simulink model "altitude_from_pitch_loop"  (Simulink 9.0)
settings: Solver=VariableStepAuto  StartTime=0.0  StopTime=100  RelTol=1e-3
InitFcn:
  | param_chap6
values from neighbouring files (symbols this model uses):
  G = getGains(P,G)    [param_chap6.m]
libraries: cstblocks x2
settings Model: SuppressorTable=22 serialization::archive 11 0 6 0 0 0 0 0  Creator=leonardopedroso  LastModifiedBy=leonardopedroso
settings DataIOCC: SaveFormat=Dataset
settings OptimizationCC: LifeSpan=auto
settings DebuggingCC: UnderspecifiedInitializationDetection=Simplified  MergeDetectMultiDrivingBlocksExec=error  SFUnexpectedBacktrackingDiag=error  SFNoUnconditionalDefaultTransitionDiag=error  SFExecutionAtInitializationDiag=warning
settings HardwareCC: ProdBitPerPointer=64  ProdBitPerSizeT=64  ProdBitPerPtrDiffT=64  ProdLargestAtomicFloat=Float  ProdIntDivRoundTo=Zero  ProdEndianess=LittleEndian  ProdWordSize=64  ProdHWDeviceType=Intel->x86-64 (Windows64)
settings ModelReferenceCC: PropagateSignalLabelsOutOfModel=on
settings CodeAppCC: StateflowObjectComments=off
settings GRTTargetCC: TargetLangStandard=C99 (ISO)
settings ConfigComp: CovMetricSettings=dwe  CovHtmlReporting=off  CovSaveCumulativeToWorkspaceVar=off  CovSaveSingleToWorkspaceVar=off  CovExternalEMLEnable=on

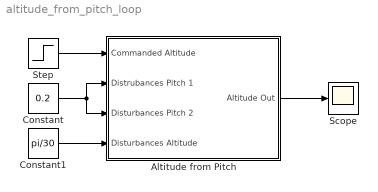
== system altitude_from_pitch_loop ==
  Altitude from Pitch : Subsystem
  Constant : Constant  Value=0.2
  Constant1 : Constant  Value=pi/30
  Scope : Scope
  Step : Step  Time=50  After=2  SampleTime=0
  wires:
  Altitude from Pitch/1(Altitude Out) -> Scope/1
  Constant/1 -> Altitude from Pitch/3(Disturbances Pitch 2), Altitude from Pitch/2(Distrubances Pitch 1)
  Constant1/1 -> Altitude from Pitch/4(Disturbances Altitude)
  Step/1 -> Altitude from Pitch/1(Commanded Altitude)

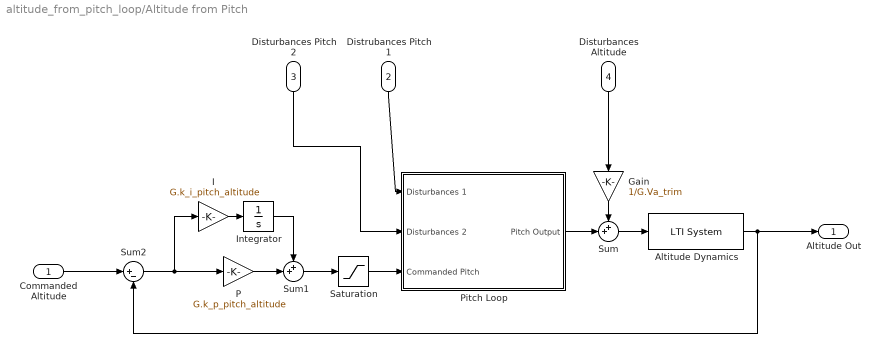
== system altitude_from_pitch_loop/Altitude from Pitch ==
  Commanded Altitude : Inport
  Distrubances Pitch 1 : Inport  Port=2
  Disturbances Pitch 2 : Inport  Port=3
  Disturbances Altitude : Inport  Port=4
  Altitude Dynamics : cstblocks/LTI System  sys=T_h_theta  IC=[]
  Gain : Gain  Gain=1/G.Va_trim
  I : Gain  Gain=G.k_i_pitch_altitude
  Integrator : Integrator
  P : Gain  Gain=G.k_p_pitch_altitude
  "Pitch Loop " : Subsystem
  Saturation : Saturate  UpperLimit=pi/4  LowerLimit=-pi/4
  Sum : Sum  Inputs=++|
  Sum1 : Sum  Inputs=++|
  Sum2 : Sum  Inputs=|+-
  Altitude Out : Outport
  wires:
  I/1 -> Integrator/1
  Sum/1 -> Altitude Dynamics/1
  Altitude Dynamics/1 -> Altitude Out/1, Sum2/2
  Integrator/1 -> Sum1/1
  P/1 -> Sum1/2
  "Pitch Loop "/1(Pitch Output) -> Sum/2
  Distrubances Pitch 1/1 -> "Pitch Loop "/1(Disturbances 1)
  Gain/1 -> Sum/1
  Sum2/1 -> P/1, I/1
  Commanded Altitude/1 -> Sum2/1
  Disturbances Pitch 2/1 -> "Pitch Loop "/2("Disturbances 2 ")
  Disturbances Altitude/1 -> Gain/1
  Sum1/1 -> Saturation/1
  Saturation/1 -> "Pitch Loop "/3(Commanded Pitch)

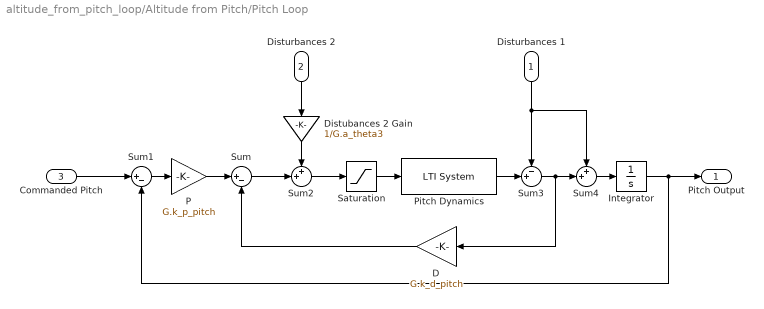
== system altitude_from_pitch_loop/Altitude from Pitch/Pitch Loop  ==
  Disturbances 1 : Inport
  "Disturbances 2 " : Inport  Port=2
  Commanded Pitch : Inport  Port=3
  D : Gain  Gain=G.k_d_pitch
  Distubances 2 Gain : Gain  Gain=1/G.a_theta3
  Integrator : Integrator
  "P " : Gain  Gain=G.k_p_pitch
  Pitch Dynamics : cstblocks/LTI System  sys=T_theta_dot_delta_e  IC=[]
  Saturation : Saturate  UpperLimit=G.delta_e_max  LowerLimit=-G.delta_a_max
  Sum : Sum  Inputs=|+-
  Sum1 : Sum  Inputs=|+-
  Sum2 : Sum  Inputs=++|
  Sum3 : Sum  Inputs=-+|
  Sum4 : Sum  Inputs=++|
  Pitch Output : Outport
  wires:
  Integrator/1 -> Pitch Output/1, Sum1/2
  Sum1/1 -> "P "/1
  Sum/1 -> Sum2/2
  Distubances 2 Gain/1 -> Sum2/1
  "Disturbances 2 "/1 -> Distubances 2 Gain/1
  Saturation/1 -> Pitch Dynamics/1
  "P "/1 -> Sum/1
  D/1 -> Sum/2
  Pitch Dynamics/1 -> Sum3/2
  Disturbances 1/1 -> Sum4/1, Sum3/1
  Sum3/1 -> D/1, Sum4/2
  Sum4/1 -> Integrator/1
  Sum2/1 -> Saturation/1
  Commanded Pitch/1 -> Sum1/1
